simulink model "SEIR1"  (R2020a)
settings: Solver=VariableStepAuto  StartTime=0.0  StopTime=300  RelTol=1e-3
values from neighbouring files (symbols this model uses):
  be = 1.860000000000000    (= 1.86)    [COVID19.m]
  ga = 1.780000000000000    (= 1.78)    [COVID19.m]
  i0 = 1/N    (= 2.77777777778e-08)    [COVID19.m]
  r0 = 0    [COVID19.m]
  s0 = 1-i0-r0    (= 0.999999972222)    [COVID19.m]
undefined symbols (not defined in the file or in its folder): al, e0
settings Model: Creator=Houda Assad

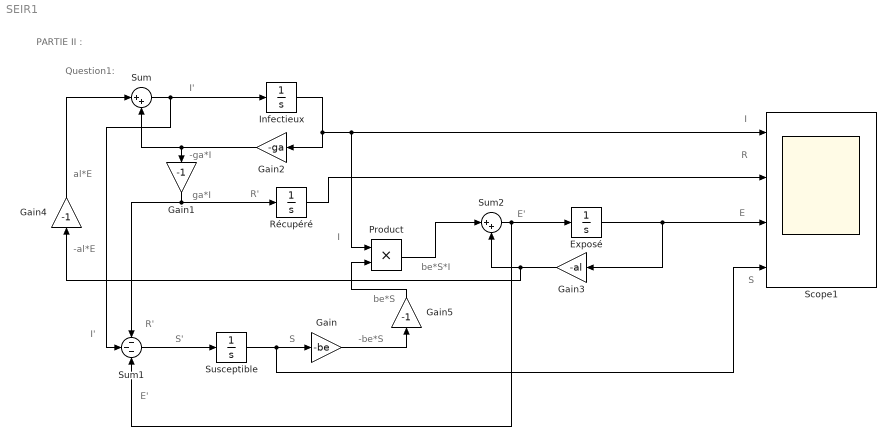
== system SEIR1 ==
  note: I'
  note: S'
  note: -al*E
  note: be*S*I
  note: I
  note: E'
  note: E
  note: Question1:
  note: ga*I
  note: S
  note: I'
  note: R'
  note: -be*S
  note: R
  note: -ga*I
  note: I
  note: S
  note: al*E
  note: R'
  note: E'
  note: PARTIE II :
  note: be*S
  Exposé : Integrator  InitialCondition=e0
  Gain : Gain  Gain=-be
  Gain1 : Gain  Gain=-1
  Gain2 : Gain  Gain=-ga
  Gain3 : Gain  Gain=-al
  Gain4 : Gain  Gain=-1
  Gain5 : Gain  Gain=-1
  Infectieux : Integrator  InitialCondition=i0
  Product : Product
  Récupéré : Integrator  InitialCondition=r0
  Scope1 : Scope  NumInputPorts=4
  Sum : Sum  Inputs=|++
  Sum1 : Sum  Inputs=---
  Sum2 : Sum  Inputs=|++
  Susceptible : Integrator  InitialCondition=s0
  wires:
  Susceptible/1 -> Scope1/4, Gain/1
  Gain2/1 -> Gain1/1, Sum/2
  Infectieux/1 -> Gain2/1, Scope1/1, Product/1
  Récupéré/1 -> Scope1/2
  Gain1/1 -> Récupéré/1, Sum1/1
  Sum1/1 -> Susceptible/1
  Sum/1 -> Sum1/2, Infectieux/1
  Exposé/1 -> Gain3/1, Scope1/3
  Gain3/1 -> Gain4/1, Sum2/2
  Sum2/1 -> Sum1/3, Exposé/1
  Product/1 -> Sum2/1
  Gain4/1 -> Sum/1
  Gain/1 -> Gain5/1
  Gain5/1 -> Product/2
